simulink model "voice_processing_mini_project"  (R2022b)
settings: Solver=VariableStepAuto  StartTime=0.0  StopTime=10.0  RelTol=1e-3
undefined symbols (not defined in the file): fdesignblkfcn, gcbh
libraries: dspsnks4 x1, dspvision x1, dspfdesign x1, dspsrcs4 x1
settings Model: Creator=prtej  LastModifiedBy=prtej

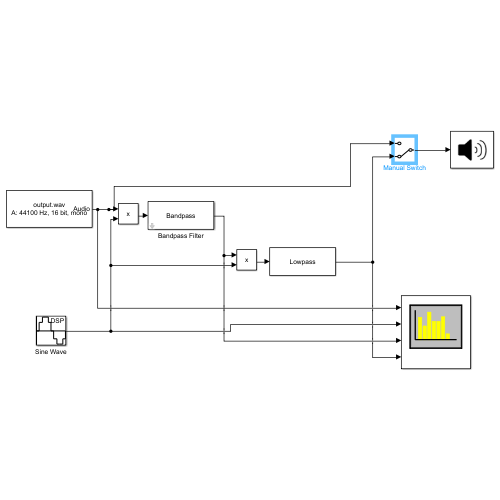
[thumbnail: Simulink's stored preview of the top-level diagram]
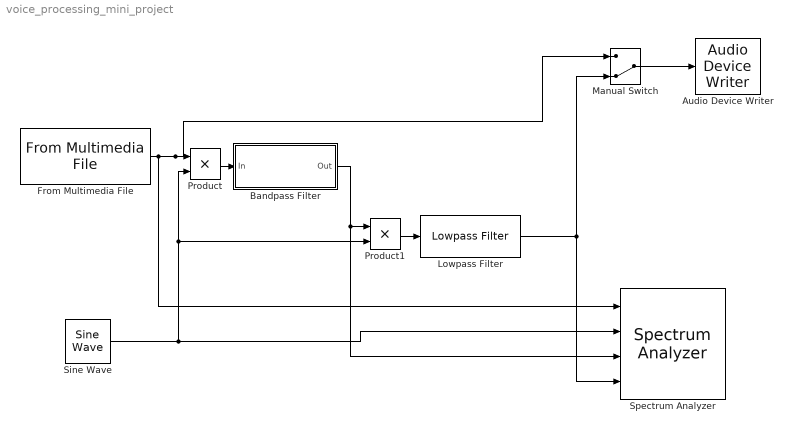
== system voice_processing_mini_project ==
  Audio Device Writer : dspsnks4/Audio Device Writer  Driver=DirectSound  Device=Default  InheritSampleRate=on  SampleRate=44100  BitDepth=16-bit integer  BufferSize=4096  NumBuffers=10  DefaultOutputChannelMapping=on  OutputChannelMapping=1:2  OutputNumUnderrunSamples=off  DriverIdx=1  DeviceWarnFlag=''
  Bandpass Filter : Subsystem  DialogController=fdesignblkfcn  InitFcn=fdesignblkfcn(gcbh, {'InitFcn'});  mask(Bandpass Filter){}
      mask help: Design a bandpass filter
      settings: CopyFcn=fdesignblkfcn(gcbh, {'CopyFcn'});
      mask Help: helpview(mapfilelocation('dsp'), 'dspbandpassfilter');
      mask Display: disp('Bandpass');
  From Multimedia File : dspvision/From Multimedia File  inputFilename=C:\Users\prtej\Downloads\output.wav  readRange=[1 Inf]  loop=on  numPlays=inf  outputStreams=Audio only  videoDataType=single  audioDataType=double  inheritSampleTime=on  userDefinedSampleTime=1/30  noAudioOutput=off  isIntensityVideo=off  fourcc=RGB  colorVideoFormat=Separate color signals  outputEOF=off  dataOrg=Column-major  audioFrameSize=1024  computeAudioFrameSize=off  outSamplingMode=Sample based
      settings: LibrarySourceBlock=audiosources/From Multimedia File
  Lowpass Filter : dspfdesign/Lowpass Filter  FilterType=FIR  DesignForMinimumOrder=on  FilterOrder=50  PassbandFrequency=19200  StopbandFrequency=20800  PassbandRipple=0.1  StopbandAttenuation=90  InheritSampleRate=off  SampleRate=44100  SimulateUsing=Interpreted execution  roundingMode=Floor  coeffsDataTypeStr=fixdt(1,16)
  Manual Switch : ManualSwitch  CurrentSetting=0
  Product : Product
  Product1 : Product
  Sine Wave : dspsrcs4/Sine Wave  Amplitude=1  Frequency=100000  Phase=0  SampleMode=Discrete  OutComplex=Real  CompMethod=Trigonometric fcn  TableSize=Speed  SampleTime=1/44100  SamplesPerFrame=1024  ResetState=Restart at time zero  OutputFrames=off  dataType=double  wordLen=16  udDataType=sfix(16)  fracBitsMode=Best precision  numFracBits=15  OutDataTypeStr=double  LastOutDataTypeStr=double
  Spectrum Analyzer : SpectrumAnalyzer  NumInputPorts=4
  wires:
  From Multimedia File/1 -> Spectrum Analyzer/1, Manual Switch/1, Product/1
  Sine Wave/1 -> Spectrum Analyzer/2, Product/2, Product1/2
  Product/1 -> Bandpass Filter/1(In)
  Bandpass Filter/1(Out) -> Spectrum Analyzer/3, Product1/1
  Product1/1 -> Lowpass Filter/1
  Manual Switch/1 -> Audio Device Writer/1
  Lowpass Filter/1 -> Spectrum Analyzer/4, Manual Switch/2

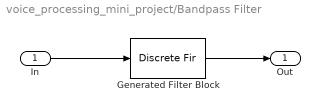
== system voice_processing_mini_project/Bandpass Filter ==
  In : Inport
  Generated Filter Block : DiscreteFir  Tag=BlockMethodSubSystem  FilterStructure=Direct form symmetric  Coefficients=[8.65773146375845293e-19 -0.000504871449931725935 -5.07955377919566214e-18 0.00097479370794624487 3.64283471851176105e-18 -0.00102067127544921911 3.70003755989170808e-19 1.83179283775204014e-17 -3.9468469351013561e-18 0.00236992554341349188 1.40488452891372709e-17 -0.0054651671644483299 -1.66460002028716477e-18 0.00755528623645561684 4.29200605938869664e-17 -0.00630393881163489583 0 4.70234310929740038e-17 -3.37124576503877518e-18 0.0109260357918192184 4.51269250684085863e-17 -0.022908621530191027 -7.20973909612515709e-17 0.029567620785256335 2.62839953959471924e-17 -0.0236377214840126845 -3.02622892972749078e-17 8.69676006573752822e-17 5.94542123367780996e-18 0.0414056386294978235 8.53295709670173523e-17 -0.0942168131611050841 -7.06433685633765601e-17 0.146763545831796571 7.49874655759525357e-17 -0.185544457384713646 -5.53605352032169945e-17 0.199831126523082048 -5.53605352032169945e-17 -0.185544457384713646 7.49874655759525357e-17 0.146763545831796571 -7.06433685633765601e-17 -0.0942168131611050841 8.53295709670173523e-17 0.0414056386294978235 5.94542123367780996e-18 8.69676006573752822e-17 -3.02622892972749078e-17 -0.0236377214840126845 2.62839953959471924e-17 0.029567620785256335 -7.20973909612515709e-17 -0.022908621530191027 4.51269250684085863e-17 0.0109260357918192184 -3.37124576503877518e-18 4.70234310929740038e-17 0 -0.00630393881163489583 4.29200605938869664e-17 0.00755528623645561684 -1.66460002028716477e-18 -0.0054651671644483299 1.40488452891372709e-17 0.00236992554341349188 -3.9468469351013561e-18 1.83179283775204014e-17 3.70003755989170808e-19 -0.00102067127544921911 3.64283471851176105e-18 0.00097479370794624487 -5.07955377919566214e-18 -0.000504871449931725935 8.65773146375845293e-19]  InputProcessing=Columns as channels (frame based)
  Out : Outport  VectorParamsAs1DForOutWhenUnconnected=off
  wires:
  In/1 -> Generated Filter Block/1
  Generated Filter Block/1 -> Out/1
